simulink model "wind_turbine_induction_generator"  (R2013a)
settings: Solver=ode3  StartTime=0.0  StopTime=30  FixedStep=0.001  RelTol=1e-3
libraries: powerlib x7, re_lib x1
settings Model: Creator=Görkem  LastModifiedBy=Görkem

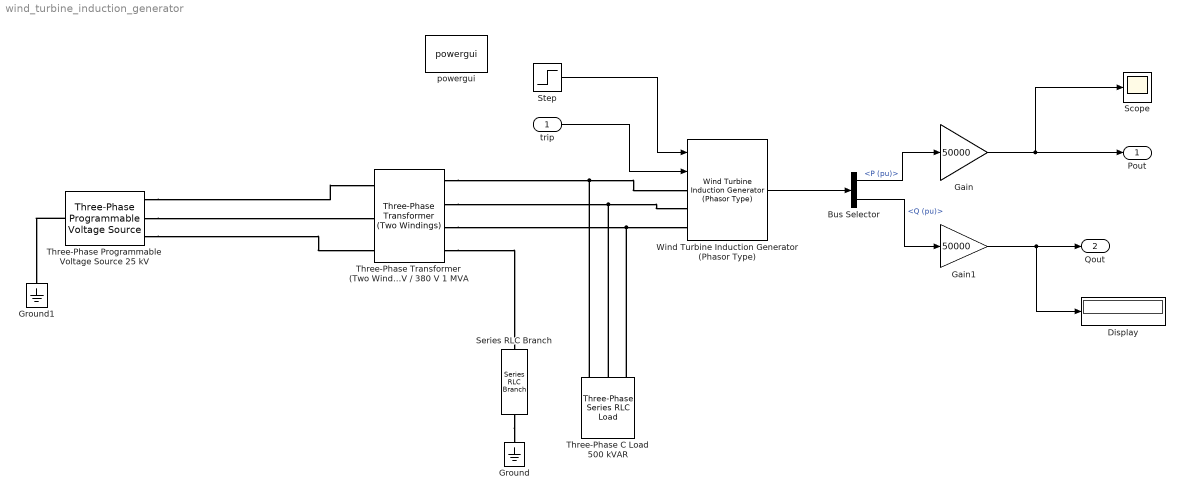
== system wind_turbine_induction_generator ==
  trip : Inport
  Bus Selector : BusSelector  OutputSignals=P (pu),Q (pu)
  Display : Display
  Gain : Gain  Gain=50000
  Gain1 : Gain  Gain=50000
  Ground : powerlib/Elements/Ground  LConnTagsString=a
  Ground1 : powerlib/Elements/Ground  LConnTagsString=a
  Scope : Scope
  Series RLC Branch : powerlib/Elements/Series RLC Branch  LConnTagsString=__new0  RConnTagsString=__new0  BranchType=R  Resistance=66  Inductance=1e-3  SetiL0=off  InitialCurrent=0  Capacitance=1e-6  Setx0=off  InitialVoltage=0  Measurements=None
  Step : Step  After=14  SampleTime=0
  Three-Phase C Load 500 kVAR : powerlib/Elements/Three-Phase Series RLC Load  LConnTagsString=A|B|C  Configuration=Delta  NominalVoltage=230  NominalFrequency=50  ActivePower=0  InductivePower=0  CapacitivePower=500000  Measurements=None  LoadType=constant Z
  Three-Phase Programmable Voltage Source 25 kV : powerlib/Electrical Sources/Three-Phase Programmable Voltage Source  PositiveSequence="[25000  0 50]"  VariationEntity=None  VariationType=Table of time-amplitude pairs  VariationTypeAlt=Step  VariationStep=0.5  VariationRate=10  VariationMagnitude=0.3  VariationFrequency=2  VariationTiming=[1 2]  VariationPhaseA=off  Amplitudes=[1 0.8 1.2 1.0]  TimeValues=[0 0.1 0.15 0.2]  HarmonicGeneration=off  HarmonicA=[3 0.2 -25 0]  HarmonicB=[2 0.15 35 2]  Timing="[0.05  3]"  BusType=swing  Pref=0  Qref=0  Qmin=-inf  Qmax=inf
  Three-Phase Transformer (Two Windings) 25 kV / 380 V 1 MVA : powerlib/Elements/Three-Phase Transformer (Two Windings)  Winding1Connection=Yg  UNITS=pu  NominalPower=[ 1000000 , 50 ]  Winding1=[25000 0.00083334 0.025]  Winding2Connection=Yn  Winding2=[380 0.00083335 0.025]  SetSaturation=off  Rm=500  Lm=Inf  Saturation=[0 0;0.0024 1.2;1 1.52]  Hysteresis=off  DataFile='hysteresis'  SetInitialFlux=off  InitialFluxes=[0.8 -0.8 0.7]  Measurements=None  MoreParameters=off  BreakLoop=off  DataType=off  TransfoNumber=1
  Wind Turbine Induction Generator (Phasor Type) : re_lib/Wind Generation/Wind Turbine Induction Generator (Phasor Type)  ShowParameters=Generator data  nom=[50000 380 50]  sta=[ 0.004843 0.1248]  rot=[ 0.004377 0.1791]  Lm=6.77  mec=[5.04 0.01 3]  init="[ -0.01,0   0,0,0   0,0,0 ]"  ExternalTm=off  DisplayTurbChar=off  pitch_angle=0  Pmec=50000  wind_base=14  P_wind_base=1  speed_nom=1  K_pitch_gain=[5 25]  pitch_max=45  pitch_rate=2
  powergui : powerlib/powergui  Priority=1  SimulationMode=Phasor  SolverType=Tustin  SampleTime=50e-6  frequency=50  SPID=off  DisableSnubberDevices=off  DisableRonSwitches=off  DisableVfSwitches=off  SwTol=0  Interpol=off  DisplayEquations=off  frequencyindice=50  Pbase=1e6  ErrMax=1e-4  Iterations=50  UnitsV=V  UnitsW=W  FunctionMessages=off  echomessages=off  HookPort=off  EnableUseOfTLC=off  x0status=blocks  RestoreLinks=warning  ResistiveCurrentMeasurement=off  Frange=[0:2:500]  Ylog=off  Xlog=on  ShowGrid=off  save=off  variable=ZData  ZoomFFT=off  StartTime=0.0  cycles=1  DisplayStyle=1  fundamental=60  FreqAxis=off  MaxFrequency=1000  frequencyindicesteady=1  RmsSteady=1  display=off  Ts=0  methode=off
  Pout : Outport
  Qout : Outport  Port=2
  wires:
  Wind Turbine Induction Generator (Phasor Type)/1 -> Bus Selector/1
  Bus Selector/1 -> Gain/1  "<P (pu)>"
  Bus Selector/2 -> Gain1/1  "<Q (pu)>"
  Gain/1 -> Pout/1, Scope/1
  Gain1/1 -> Display/1, Qout/1
  trip/1 -> Wind Turbine Induction Generator (Phasor Type)/2
  Step/1 -> Wind Turbine Induction Generator (Phasor Type)/1
  connections:
  Three-Phase Transformer (Two Windings) 25 kV / 380 V 1 MVA/RConn4 -- Series RLC Branch/LConn1
  Series RLC Branch/RConn1 -- Ground/LConn1
  Three-Phase Programmable Voltage Source 25 kV/LConn1 -- Ground1/LConn1
  Three-Phase Programmable Voltage Source 25 kV/RConn1 -- Three-Phase Transformer (Two Windings) 25 kV / 380 V 1 MVA/LConn1
  Three-Phase Programmable Voltage Source 25 kV/RConn2 -- Three-Phase Transformer (Two Windings) 25 kV / 380 V 1 MVA/LConn2
  Three-Phase Programmable Voltage Source 25 kV/RConn3 -- Three-Phase Transformer (Two Windings) 25 kV / 380 V 1 MVA/LConn3
  Three-Phase Transformer (Two Windings) 25 kV / 380 V 1 MVA/RConn1 -- Three-Phase C Load 500 kVAR/LConn1 -- Wind Turbine Induction Generator (Phasor Type)/LConn1
  Three-Phase Transformer (Two Windings) 25 kV / 380 V 1 MVA/RConn2 -- Three-Phase C Load 500 kVAR/LConn2 -- Wind Turbine Induction Generator (Phasor Type)/LConn2
  Three-Phase Transformer (Two Windings) 25 kV / 380 V 1 MVA/RConn3 -- Three-Phase C Load 500 kVAR/LConn3 -- Wind Turbine Induction Generator (Phasor Type)/LConn3
